simulink model "Nonlinear_system"  (Simulink 8.1)
settings: Solver=ode45  StartTime=0.0  StopTime=0.8  FixedStep=0.000005  MaxStep=5e-4  MinStep=5e-6  RelTol=1e-3
settings Model: Creator=mainster  LastModifiedBy=mainster

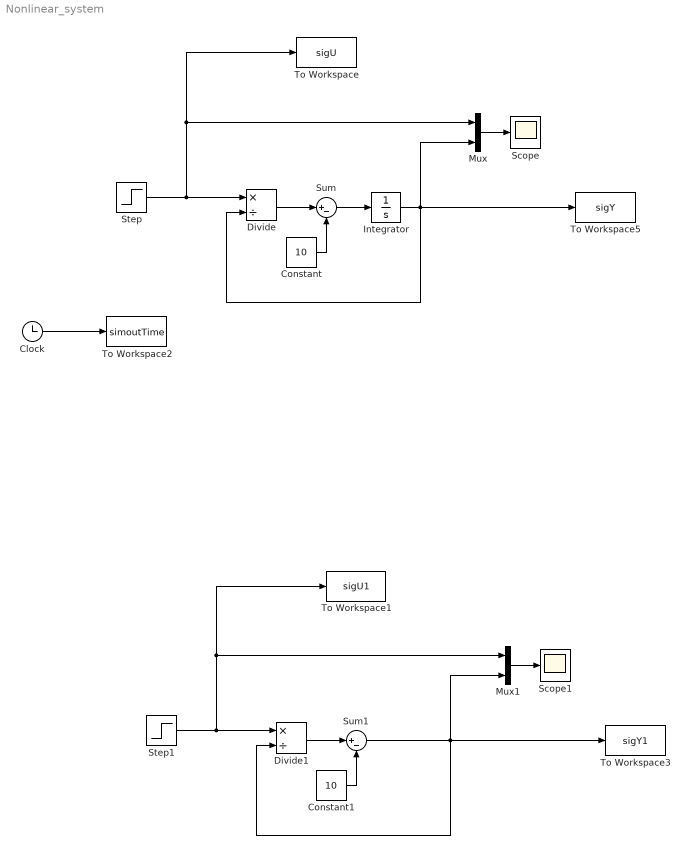
== system Nonlinear_system ==
  Clock : Clock
  Constant : Constant  Value=10
  Constant1 : Constant  Value=10
  Divide : Product  Inputs=*/
  Divide1 : Product  Inputs=*/
  Integrator : Integrator  InitialCondition=2
  Mux : Mux  Inputs=2
  Mux1 : Mux  Inputs=2
  Scope : Scope
  Scope1 : Scope
  Step : Step  Time=0.1  SampleTime=0
  Step1 : Step  Time=0.1  After=2  SampleTime=0
  Sum : Sum  Inputs=|+-
  Sum1 : Sum  Inputs=|+-
  To Workspace : ToWorkspace  VariableName=sigU  SampleTime=-1  SaveFormat=Structure
  To Workspace1 : ToWorkspace  VariableName=sigU1  SampleTime=-1  SaveFormat=Structure
  To Workspace2 : ToWorkspace  VariableName=simoutTime  SampleTime=-1  SaveFormat=Structure
  To Workspace3 : ToWorkspace  VariableName=sigY1  SampleTime=-1  SaveFormat=Structure
  To Workspace5 : ToWorkspace  VariableName=sigY  SampleTime=-1  SaveFormat=Structure
  wires:
  Clock/1 -> To Workspace2/1
  Step/1 -> Divide/1, Mux/1, To Workspace/1
  Divide/1 -> Sum/1
  Constant/1 -> Sum/2
  Sum/1 -> Integrator/1
  Integrator/1 -> Divide/2, Mux/2, To Workspace5/1
  Mux/1 -> Scope/1
  Step1/1 -> Divide1/1, Mux1/1, To Workspace1/1
  Divide1/1 -> Sum1/1
  Constant1/1 -> Sum1/2
  Sum1/1 -> Divide1/2, Mux1/2, To Workspace3/1
  Mux1/1 -> Scope1/1
